simulink model "sampleModel2041"  (R2023a)
settings: Solver=VariableStepAuto  StartTime=0.0  StopTime=10.0  RelTol=1e-3
libraries: hdlsllib x8, simulink x1
settings Model: Creator=user1  LastModifiedBy=user1

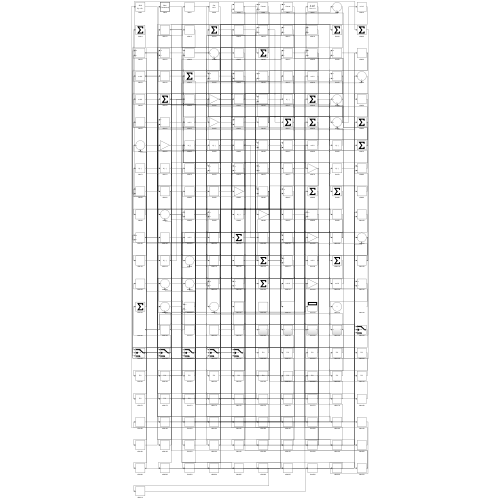
[thumbnail: Simulink's stored preview of the top-level diagram]
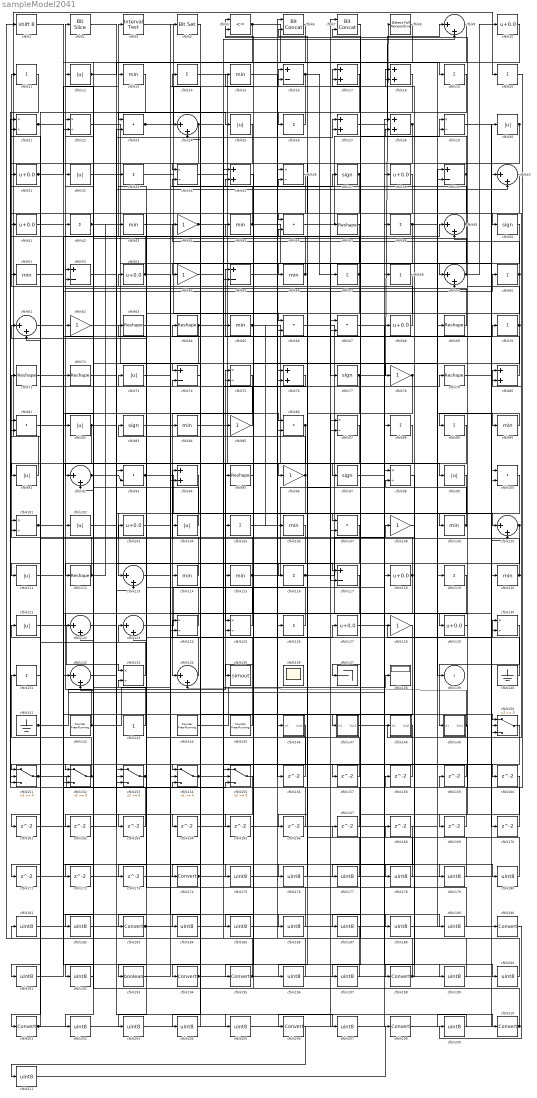
== system sampleModel2041 ==
  cfblk1 : ArithShift  BitShiftNumber=8
  cfblk{10,31,38,41,53,68,103,118,127,129} (10 alike) : Bias  Bias=0.0  SaturateOnIntegerOverflow=off
  cfblk{23,46,66..67,81,86,93,100,107} (9 alike) : DotProduct  OutDataTypeStr=Inherit: Inherit via internal rule
  cfblk{21..22,29,34,36,75,87,98,101,124..125,130,133} (13 alike) : Product  Inputs=*/  RndMeth=Zero  SaturateOnIntegerOverflow=on
  cfblk{12,25,30,32,73,82,91,99,102,104,111,121} (12 alike) : Abs  SaturateOnIntegerOverflow=off
  cfblk{11,14,19..20,26,33,42,48,57..58,60,70,88..89,105,116,119,126,131} (19 alike) : Sum  Inputs=+
  cfblk{13,15,43,45,51,56,65,84,90,106,109,114..115,120} (14 alike) : MinMax
  cfblk{44,54,62,78,85,96,108,128} (8 alike) : Gain
  cfblk{9,24,40,49,59,61,92,110,113,122..123,132,134} (13 alike) : Sum  Inputs=|++
  cfblk{47,63..64,69,71..72,79,95,112} (9 alike) : Reshape
  cfblk{16,39,52,55,74,117} (6 alike) : Sum  Inputs=+-
  cfblk135 : ToWorkspace  VariableName=simout  SaveFormat=Timeseries  SampleTime=-1
  cfblk136 : Scope
      settings: Floating=on
  cfblk137 : Terminator
  cfblk138 : Display
  cfblk140 : Ground
  cfblk141 : Ground
  cfblk142 : hdlsllib/Sources/Counter Free-Running  NumBits=16  tsamp=-1
  cfblk143 : Constant  SampleTime=-1
  cfblk144 : hdlsllib/Sources/Counter Free-Running  NumBits=16  tsamp=-1
  cfblk145 : hdlsllib/Sources/Counter Free-Running  NumBits=16  tsamp=-1
  cfblk146 : Subsystem
      settings: LibrarySourceBlock=|
      | hdlsllib/Ports &
      | Subsystems/Subsystem
  cfblk147 : Subsystem
      settings: LibrarySourceBlock=|
      | hdlsllib/Ports &
      | Subsystems/Subsystem
  cfblk148 : Subsystem
      settings: LibrarySourceBlock=|
      | hdlsllib/Ports &
      | Subsystems/Subsystem
  cfblk149 : Subsystem
      settings: LibrarySourceBlock=|
      | hdlsllib/Ports &
      | Subsystems/Subsystem
  cfblk{150..155} (6 alike) : Switch  SaturateOnIntegerOverflow=off  InputSameDT=off
  cfblk{156..173} (18 alike) : Delay  SampleTime=1
  cfblk{17..18,27..28,35,76,80,94} (8 alike) : Sum
  cfblk{174,183,190,194..195,198,201,206,208,210} (10 alike) : DataTypeConversion  SaturateOnIntegerOverflow=off  RndMeth=Floor
  cfblk{175..182,184..189,191..192,196..197,199..200,202..205,207,209,211} (27 alike) : DataTypeConversion  OutDataTypeStr=uint8  SaturateOnIntegerOverflow=off  RndMeth=Floor
  cfblk193 : DataTypeConversion  OutDataTypeStr=boolean  SaturateOnIntegerOverflow=off  RndMeth=Floor
  cfblk2 : hdlsllib/Logic and Bit Operations/Bit Slice  lidx=7  ridx=0
  cfblk3 : hdlsllib/Logic and Bit Operations/Interval Test  IntervalClosedRight=on  uplimit=0.5  IntervalClosedLeft=on  lowlimit=-0.5  OutDataTypeStr=boolean
  cfblk{37,50,77,83,97} (5 alike) : Signum
  cfblk4 : simulink/Logic and Bit Operations/Bit Set  iBit=0
      settings: LibrarySourceBlock=|
      | hdlsllib/Logic and Bit
      | Operations/Bit Set
  cfblk5 : RelationalOperator  Operator=<=  OutDataTypeStr=boolean  InputSameDT=off
  cfblk6 : hdlsllib/Logic and Bit Operations/Bit Concat  numInputs=2
  cfblk7 : hdlsllib/Logic and Bit Operations/Bit Concat  numInputs=2
  cfblk8 : hdlsllib/Logic and Bit Operations/Detect Fall Nonpositive  vinit=0  OutDataTypeStr=boolean
  cfblk139 : Outport  VectorParamsAs1DForOutWhenUnconnected=off
  wires:
  cfblk69/1 -> cfblk2/1
  cfblk81/1 -> cfblk52/1
  cfblk143/1 -> cfblk42/1
  cfblk3/1 -> cfblk66/1
  cfblk66/1 -> cfblk129/1
  cfblk110/1 -> cfblk122/2, cfblk178/1
  cfblk91/1 -> cfblk20/1
  cfblk127/1 -> cfblk130/1
  cfblk82/1 -> cfblk113/2, cfblk161/1
  cfblk130/1 -> cfblk149/1(In1)
  cfblk16/1 -> cfblk57/1, cfblk152/2
  cfblk50/1 -> cfblk96/1
  cfblk142/1 -> cfblk52/2, cfblk127/1
  cfblk27/1 -> cfblk9/1
  cfblk53/1 -> cfblk3/1, cfblk86/1
  cfblk68/1 -> cfblk11/1
  cfblk14/1 -> cfblk99/1
  cfblk125/1 -> cfblk41/1
  cfblk46/1 -> cfblk29/1
  cfblk114/1 -> cfblk71/1
  cfblk141/1 -> cfblk75/1, cfblk28/1
  cfblk85/1 -> cfblk51/1
  cfblk15/1 -> cfblk126/1
  cfblk35/1 -> cfblk195/1
  cfblk124/1 -> cfblk73/1
  cfblk56/1 -> cfblk54/1, cfblk15/1
  cfblk118/1 -> cfblk12/1, cfblk153/3, cfblk92/2
  cfblk57/1 -> cfblk32/1, cfblk95/1
  cfblk65/1 -> cfblk118/1, cfblk106/1
  cfblk122/1 -> cfblk70/1
  cfblk79/1 -> cfblk30/1
  cfblk92/1 -> cfblk93/2, cfblk117/1
  cfblk77/1 -> cfblk8/1, cfblk116/1
  cfblk42/1 -> cfblk85/1, cfblk40/2
  cfblk83/1 -> cfblk134/1
  cfblk22/1 -> cfblk155/1
  cfblk147/1(Out1) -> cfblk50/1
  cfblk33/1 -> cfblk59/1
  cfblk34/1 -> cfblk119/1
  cfblk75/1 -> cfblk84/1
  cfblk17/1 -> cfblk74/1
  cfblk48/1 -> cfblk56/1, cfblk90/1
  cfblk70/1 -> cfblk5/1, cfblk49/2, cfblk165/1
  cfblk95/1 -> cfblk5/2
  cfblk74/1 -> cfblk114/1
  cfblk49/1 -> cfblk24/2, cfblk166/1
  cfblk21/1 -> cfblk86/2, cfblk179/1
  cfblk104/1 -> cfblk62/1
  cfblk153/1 -> cfblk83/1, cfblk33/1
  cfblk109/1 -> cfblk107/1, cfblk46/2
  cfblk51/1 -> cfblk150/1
  cfblk87/1 -> cfblk201/1
  cfblk134/1 -> cfblk61/1
  cfblk116/1 -> cfblk88/1, cfblk148/1(In1)
  cfblk115/1 -> cfblk94/1, cfblk47/1, cfblk152/3
  cfblk47/1 -> cfblk66/2
  cfblk4/1 -> cfblk194/1
  cfblk88/1 -> cfblk104/1
  cfblk8/1 -> cfblk92/1
  cfblk80/1 -> cfblk55/1
  cfblk28/1 -> cfblk111/1, cfblk46/1
  cfblk6/1 -> cfblk174/1
  cfblk120/1 -> cfblk61/2, cfblk80/1
  cfblk61/1 -> cfblk72/1
  cfblk23/1 -> cfblk16/1, cfblk17/2
  cfblk86/1 -> cfblk125/1, cfblk193/1
  cfblk76/1 -> cfblk75/2
  cfblk25/1 -> cfblk55/2
  cfblk123/1 -> cfblk68/1
  cfblk126/1 -> cfblk64/1
  cfblk9/1 -> cfblk34/1
  cfblk38/1 -> cfblk112/1
  cfblk154/1 -> cfblk138/1, cfblk9/2
  cfblk99/1 -> cfblk113/1
  cfblk5/1 -> cfblk139/1, cfblk164/1
  cfblk26/1 -> cfblk23/1
  cfblk30/1 -> cfblk101/2, cfblk157/1
  cfblk44/1 -> cfblk120/1, cfblk18/2
  cfblk119/1 -> cfblk135/1
  cfblk112/1 -> cfblk81/1, cfblk43/1, cfblk162/1
  cfblk144/1 -> cfblk48/1
  cfblk140/1 -> cfblk53/1
  cfblk2/1 -> cfblk150/2
  cfblk106/1 -> cfblk152/1
  cfblk45/1 -> cfblk77/1, cfblk34/2
  cfblk121/1 -> cfblk133/1
  cfblk43/1 -> cfblk69/1
  cfblk32/1 -> cfblk76/2
  cfblk113/1 -> cfblk27/1
  cfblk24/1 -> cfblk82/1, cfblk160/1
  cfblk31/1 -> cfblk13/1, cfblk97/1
  cfblk19/1 -> cfblk154/1
  cfblk100/1 -> cfblk183/1
  cfblk36/1 -> cfblk105/1
  cfblk84/1 -> cfblk79/1
  cfblk145/1 -> cfblk124/1
  cfblk98/1 -> cfblk198/1
  cfblk63/1 -> cfblk24/1
  cfblk37/1 -> cfblk173/1, cfblk185/1
  cfblk151/1 -> cfblk60/1, cfblk155/3, cfblk154/3
  cfblk18/1 -> cfblk26/1
  cfblk93/1 -> cfblk109/1, cfblk37/1
  cfblk55/1 -> cfblk110/1
  cfblk129/1 -> cfblk29/2
  cfblk60/1 -> cfblk94/2, cfblk44/1, cfblk196/1
  cfblk133/1 -> cfblk21/2
  cfblk11/1 -> cfblk151/3
  cfblk111/1 -> cfblk49/1
  cfblk152/1 -> cfblk131/1, cfblk172/1
  cfblk149/1(Out1) -> cfblk134/2, cfblk169/1
  cfblk108/1 -> cfblk18/1
  cfblk73/1 -> cfblk130/2
  cfblk59/1 -> cfblk22/1, cfblk10/1, cfblk28/2
  cfblk78/1 -> cfblk137/1, cfblk117/2
  cfblk131/1 -> cfblk31/1
  cfblk94/1 -> cfblk124/2
  cfblk39/1 -> cfblk147/1(In1), cfblk17/1, cfblk81/2
  cfblk40/1 -> cfblk91/1
  cfblk62/1 -> cfblk146/1(In1)
  cfblk101/1 -> cfblk45/1, cfblk65/1
  cfblk10/1 -> cfblk22/2
  cfblk12/1 -> cfblk19/1, cfblk25/1
  cfblk148/1(Out1) -> cfblk154/2
  cfblk52/1 -> cfblk27/2
  cfblk64/1 -> cfblk78/1, cfblk122/1
  cfblk96/1 -> cfblk63/1, cfblk153/2
  cfblk90/1 -> cfblk89/1
  cfblk105/1 -> cfblk156/1
  cfblk156/1 -> cfblk123/2
  cfblk157/1 -> cfblk76/1
  cfblk158/1 -> cfblk151/1
  cfblk20/1 -> cfblk159/1
  cfblk159/1 -> cfblk151/2
  cfblk161/1 -> cfblk93/1
  cfblk162/1 -> cfblk23/2
  cfblk150/1 -> cfblk163/1
  cfblk163/1 -> cfblk153/1
  cfblk164/1 -> cfblk39/2
  cfblk165/1 -> cfblk107/2
  cfblk166/1 -> cfblk21/1
  cfblk167/1 -> cfblk101/1
  cfblk169/1 -> cfblk125/2
  cfblk29/1 -> cfblk170/1
  cfblk170/1 -> cfblk59/2
  cfblk13/1 -> cfblk171/1
  cfblk171/1 -> cfblk155/2
  cfblk172/1 -> cfblk16/2
  cfblk173/1 -> cfblk133/2
  cfblk174/1 -> cfblk110/2, cfblk38/1
  cfblk72/1 -> cfblk175/1
  cfblk175/1 -> cfblk6/1
  cfblk54/1 -> cfblk176/1
  cfblk176/1 -> cfblk6/2
  cfblk7/1 -> cfblk177/1
  cfblk177/1 -> cfblk36/2
  cfblk178/1 -> cfblk7/1
  cfblk179/1 -> cfblk7/2
  cfblk67/1 -> cfblk180/1
  cfblk180/1 -> cfblk158/1
  cfblk181/1 -> cfblk67/1
  cfblk117/1 -> cfblk182/1
  cfblk182/1 -> cfblk67/2
  cfblk183/1 -> cfblk39/1, cfblk58/1
  cfblk107/1 -> cfblk184/1
  cfblk184/1 -> cfblk100/1
  cfblk185/1 -> cfblk100/2
  cfblk1/1 -> cfblk186/1
  cfblk186/1 -> cfblk123/1
  cfblk160/1 -> cfblk187/1
  cfblk187/1 -> cfblk1/1
  cfblk103/1 -> cfblk188/1
  cfblk188/1 -> cfblk108/1
  cfblk41/1 -> cfblk189/1
  cfblk189/1 -> cfblk103/1
  cfblk146/1(Out1) -> cfblk191/1
  cfblk191/1 -> cfblk132/1
  cfblk155/1 -> cfblk192/1
  cfblk192/1 -> cfblk132/2
  cfblk193/1 -> cfblk4/1
  cfblk194/1 -> cfblk80/2, cfblk14/1
  cfblk195/1 -> cfblk150/3, cfblk121/1
  cfblk196/1 -> cfblk35/1
  cfblk168/1 -> cfblk197/1
  cfblk197/1 -> cfblk35/2
  cfblk198/1 -> cfblk168/1, cfblk167/1, cfblk36/1
  cfblk97/1 -> cfblk199/1
  cfblk199/1 -> cfblk98/1
  cfblk71/1 -> cfblk200/1
  cfblk200/1 -> cfblk98/2
  cfblk201/1 -> cfblk181/1, cfblk40/1
  cfblk89/1 -> cfblk202/1
  cfblk202/1 -> cfblk87/1
  cfblk58/1 -> cfblk203/1
  cfblk203/1 -> cfblk87/2
  cfblk128/1 -> cfblk204/1
  cfblk204/1 -> cfblk74/2
  cfblk102/1 -> cfblk205/1
  cfblk205/1 -> cfblk128/1
  cfblk132/1 -> cfblk207/1
  cfblk207/1 -> cfblk190/1
  cfblk208/1 -> cfblk210/1
  cfblk190/1 -> cfblk209/1
  cfblk209/1 -> cfblk206/1
  cfblk210/1 -> cfblk102/1, cfblk115/1
  cfblk206/1 -> cfblk211/1
  cfblk211/1 -> cfblk208/1

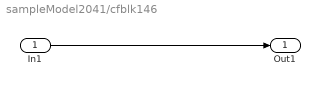
== system sampleModel2041/cfblk146 ==
  In1 : Inport
  Out1 : Outport
  wires:
  In1/1 -> Out1/1

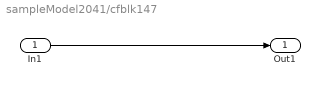
== system sampleModel2041/cfblk147 ==
  In1 : Inport
  Out1 : Outport
  wires:
  In1/1 -> Out1/1

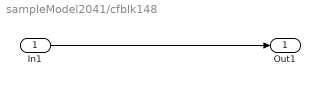
== system sampleModel2041/cfblk148 ==
  In1 : Inport
  Out1 : Outport
  wires:
  In1/1 -> Out1/1

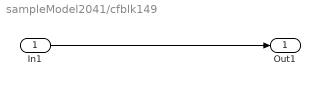
== system sampleModel2041/cfblk149 ==
  In1 : Inport
  Out1 : Outport
  wires:
  In1/1 -> Out1/1
